simulink model "AsmaroProject2"  (R2017b)
settings: Solver=VariableStepAuto  StartTime=0.0  StopTime=inf  RelTol=1e-3
libraries: DigiConLib x4, realtime_pacer_lib x1
settings Model: Creator=Danny  LastModifiedBy=Danny
settings DebuggingCC: SFInvalidInputDataAccessInChartInitDiag=none

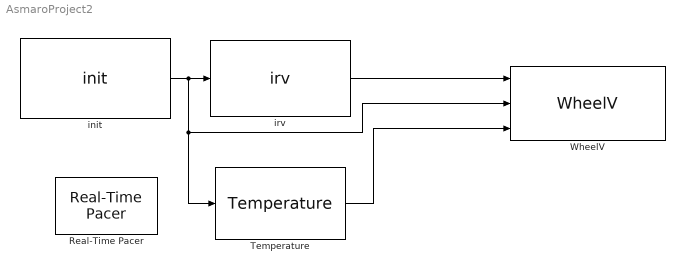
== system AsmaroProject2 ==
  Real-Time Pacer : realtime_pacer_lib/Real-Time Pacer  simTimePerRealTime=0.5
  Temperature : DigiConLib/Temperature
  WheelV : DigiConLib/WheelV
  init : DigiConLib/init
  irv : DigiConLib/irv
  wires:
  init/1 -> WheelV/2, Temperature/1, irv/1
  irv/1 -> WheelV/1
  Temperature/1 -> WheelV/3
